simulink model "Proyecto_labII_V1"  (R2025b)
settings: Solver=VariableStepAuto  StartTime=0.0  StopTime=1  RelTol=1e-3
undefined symbols (not defined in the file): gray
libraries: commsequence2 x2, commcrc2 x2, commchan3 x1, commsink2 x1, commcnvcod2 x1
settings Model: Creator=juand  LastModifiedBy=juand

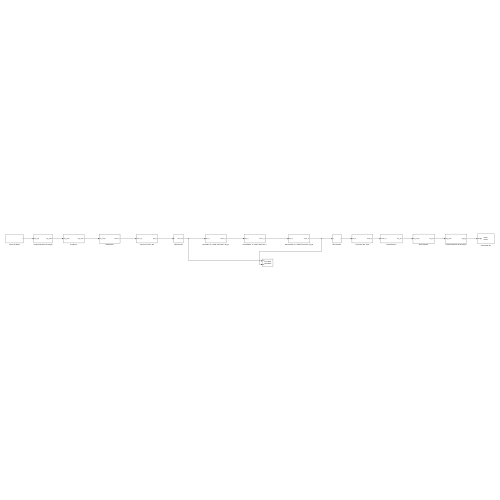
[thumbnail: Simulink's stored preview of the top-level diagram]
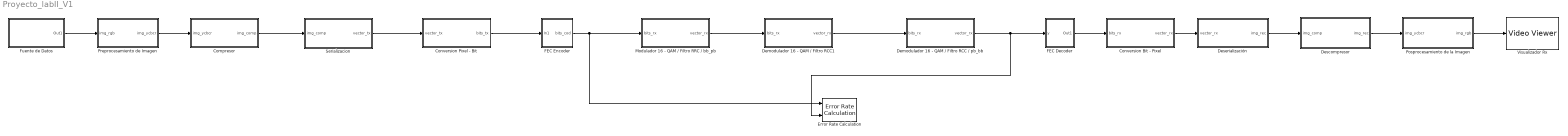
== system Proyecto_labII_V1 ==
  Compresor : Subsystem
  Conversion Bit - Pixel : Subsystem
  Conversion Pixel - Bit : Subsystem
  Demodulador 16 - QAM / Filtro RCC / pb_bb : Subsystem
  Demodulador 16 - QAM / Filtro RCC1 : Subsystem
  Descompresor : Subsystem
  Deserialización : Subsystem
  Error Rate Calculation : commsink2/Error Rate Calculation  N=0  st_delay=0  cp_mode=Entire frame  subframe=[]  PMode=Workspace  WsName=ber_out  RsMode2=off  stop=off  numErr=100  maxBits=1e6
  "FEC Decoder " : Subsystem
  FEC Encoder : Subsystem
  Fuente de Datos : Subsystem
  Modulador 16 - QAM / Filtro RRC / bb_pb : Subsystem
  Posprocesamiento de la Imagen : Subsystem
  Preprocesamiento de Imagen : Subsystem
  Serializacion : Subsystem
  Visualizador Rx : VideoViewer  colormapValue=gray(256)  FigPos=[21 783 890 663]  OpenAtMdlStart=off
  wires:
  Fuente de Datos/1(Out1) -> Preprocesamiento de Imagen/1(img_rgb)
  Preprocesamiento de Imagen/1(img_ycbcr) -> Compresor/1(img_ycbcr)
  Compresor/1(img_comp) -> Serializacion/1(img_comp)
  Deserialización/1(img_rec) -> Descompresor/1(img_comp)
  Descompresor/1(img_rec) -> Posprocesamiento de la Imagen/1(img_ycbcr)
  Serializacion/1(vector_tx) -> Conversion Pixel - Bit/1(vector_tx)
  Conversion Bit - Pixel/1(vector_rx) -> Deserialización/1(vector_rx)
  Posprocesamiento de la Imagen/1(img_rgb) -> Visualizador Rx/1
  Conversion Pixel - Bit/1(bits_tx) -> FEC Encoder/1(In1)
  "FEC Decoder "/1(Out1) -> Conversion Bit - Pixel/1(bits_rx)
  Demodulador 16 - QAM / Filtro RCC / pb_bb/1(vector_rx) -> Error Rate Calculation/2, "FEC Decoder "/1(y)
  FEC Encoder/1(bits_cod) -> Error Rate Calculation/1, Modulador 16 - QAM / Filtro RRC / bb_pb/1(bits_rx)
  Modulador 16 - QAM / Filtro RRC / bb_pb/1(vector_rx) -> Demodulador 16 - QAM / Filtro RCC1/1(bits_rx)
  Demodulador 16 - QAM / Filtro RCC1/1(vector_rx) -> Demodulador 16 - QAM / Filtro RCC / pb_bb/1(bits_rx)

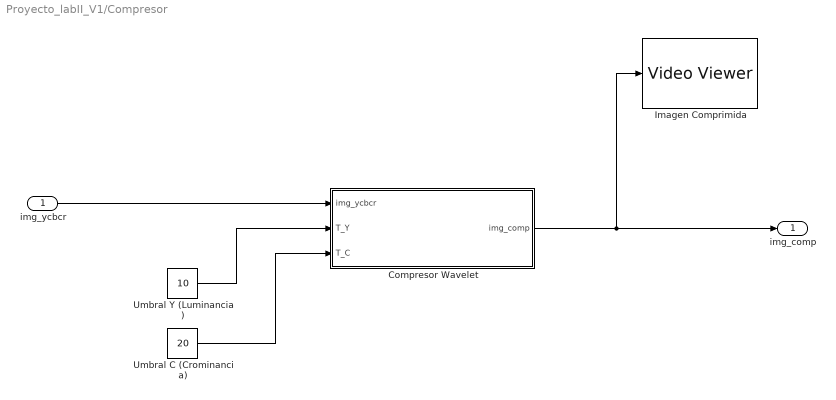
== system Proyecto_labII_V1/Compresor ==
  img_ycbcr : Inport
  Compresor Wavelet : MATLAB Function  TreatAsAtomicUnit=on
  Imagen Comprimida : VideoViewer  colormapValue=gray(256)  FigPos=[1 910 1536 813]  OpenAtMdlStart=off
  Umbral C (Crominancia) : Constant  Value=20
  Umbral Y (Luminancia) : Constant  Value=10
  img_comp : Outport
  wires:
  Compresor Wavelet/1(img_comp) -> Imagen Comprimida/1, img_comp/1
  Umbral C (Crominancia)/1 -> Compresor Wavelet/3(T_C)
  Umbral Y (Luminancia)/1 -> Compresor Wavelet/2(T_Y)
  img_ycbcr/1 -> Compresor Wavelet/1(img_ycbcr)

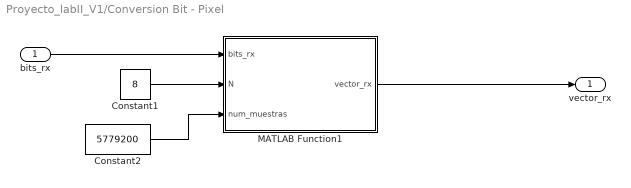
== system Proyecto_labII_V1/Conversion Bit - Pixel ==
  bits_rx : Inport
  Constant1 : Constant  Value=8
  Constant2 : Constant  Value=5779200
  MATLAB Function1 : MATLAB Function  TreatAsAtomicUnit=on
  vector_rx : Outport
  wires:
  Constant1/1 -> MATLAB Function1/2(N)
  bits_rx/1 -> MATLAB Function1/1(bits_rx)
  Constant2/1 -> MATLAB Function1/3(num_muestras)
  MATLAB Function1/1(vector_rx) -> vector_rx/1

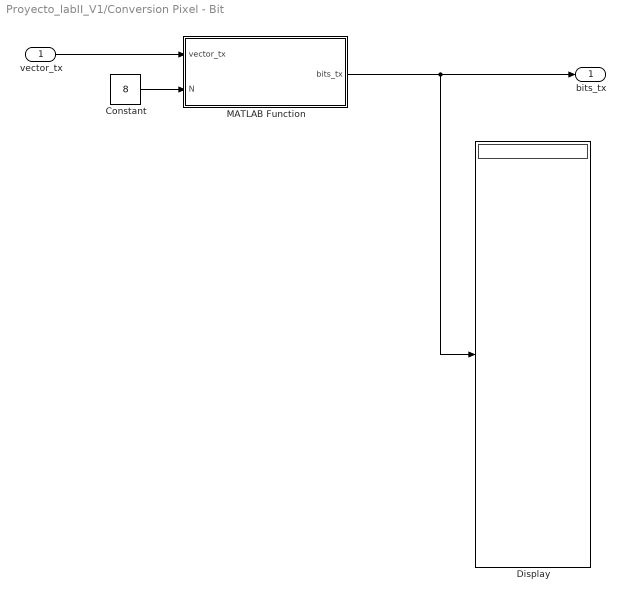
== system Proyecto_labII_V1/Conversion Pixel - Bit ==
  vector_tx : Inport
  Constant : Constant  Value=8
  Display : Display
  MATLAB Function : MATLAB Function  TreatAsAtomicUnit=on
  bits_tx : Outport
  wires:
  Constant/1 -> MATLAB Function/2(N)
  vector_tx/1 -> MATLAB Function/1(vector_tx)
  MATLAB Function/1(bits_tx) -> Display/1, bits_tx/1

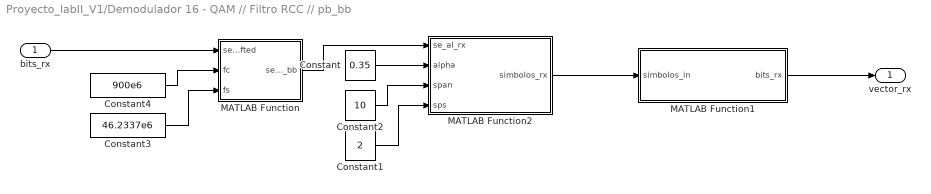
== system Proyecto_labII_V1/Demodulador 16 - QAM // Filtro RCC // pb_bb ==
  bits_rx : Inport
  Constant : Constant  Value=0.35
  Constant1 : Constant  Value=2
  Constant2 : Constant  Value=10
  Constant3 : Constant  Value=46.2337e6
  Constant4 : Constant  Value=900e6
  MATLAB Function : MATLAB Function  TreatAsAtomicUnit=on
  MATLAB Function1 : MATLAB Function  TreatAsAtomicUnit=on
  MATLAB Function2 : MATLAB Function  TreatAsAtomicUnit=on
  vector_rx : Outport
  wires:
  MATLAB Function1/1(bits_rx) -> vector_rx/1
  MATLAB Function2/1(simbolos_rx) -> MATLAB Function1/1(simbolos_in)
  bits_rx/1 -> MATLAB Function/1(senal_shifted)
  Constant1/1 -> MATLAB Function2/4(sps)
  Constant/1 -> MATLAB Function2/2(alpha)
  Constant2/1 -> MATLAB Function2/3(span)
  MATLAB Function/1(senal_bb) -> MATLAB Function2/1(se_al_rx)
  Constant4/1 -> MATLAB Function/2(fc)
  Constant3/1 -> MATLAB Function/3(fs)

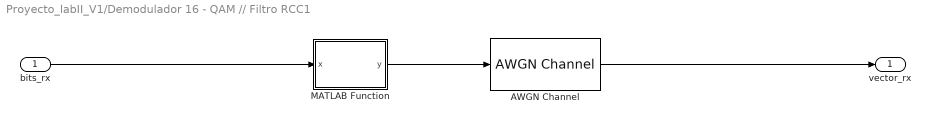
== system Proyecto_labII_V1/Demodulador 16 - QAM // Filtro RCC1 ==
  bits_rx : Inport
  AWGN Channel : commchan3/AWGN Channel  LegacyMode=off  NoiseMethod="Signal to noise ratio  (SNR)"  noiseMode="Signal to noise ratio  (SNR)"  EbNo=EbN0  EsNo=10  SNR=10  BitsPerSymbol=4  SignalPower=1  SpecifySymbolPeriod=off  SamplesPerSymbol=10  SymbolPeriod=1  VarianceSource=Parameter  Variance=1  RandomStream=Global stream  Seed=67  SimulateUsing=Code generation
  MATLAB Function : MATLAB Function  TreatAsAtomicUnit=on
  vector_rx : Outport
  wires:
  AWGN Channel/1 -> vector_rx/1
  MATLAB Function/1(y) -> AWGN Channel/1
  bits_rx/1 -> MATLAB Function/1(x)

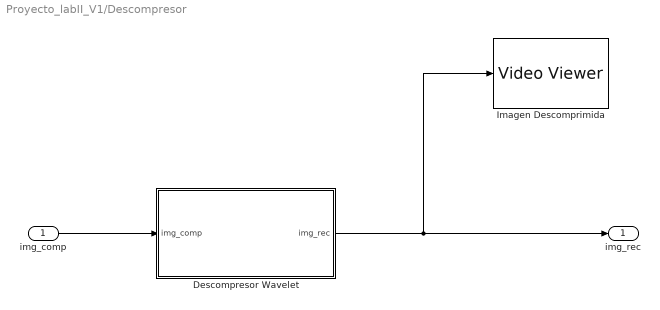
== system Proyecto_labII_V1/Descompresor ==
  img_comp : Inport
  Descompresor Wavelet : MATLAB Function  TreatAsAtomicUnit=on
  Imagen Descomprimida : VideoViewer  colormapValue=gray(256)  FigPos=[1 910 1536 813]  OpenAtMdlStart=off
  img_rec : Outport
  wires:
  Descompresor Wavelet/1(img_rec) -> Imagen Descomprimida/1, img_rec/1
  img_comp/1 -> Descompresor Wavelet/1(img_comp)

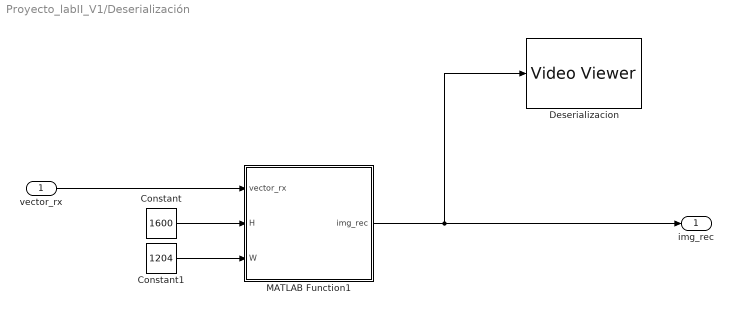
== system Proyecto_labII_V1/Deserialización ==
  vector_rx : Inport
  Constant : Constant  Value=1600
  Constant1 : Constant  Value=1204
  Deserializacion : VideoViewer  FigPos=[559 631 418 304]  OpenAtMdlStart=off
  MATLAB Function1 : MATLAB Function  TreatAsAtomicUnit=on
  img_rec : Outport
  wires:
  Constant1/1 -> MATLAB Function1/3(W)
  Constant/1 -> MATLAB Function1/2(H)
  MATLAB Function1/1(img_rec) -> Deserializacion/1, img_rec/1
  vector_rx/1 -> MATLAB Function1/1(vector_rx)

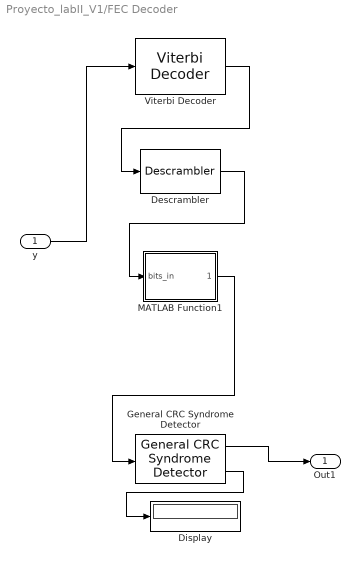
== system Proyecto_labII_V1/FEC Decoder  ==
  y : Inport
  Descrambler : commsequence2/Descrambler  M=2  poly='1 + z^-3 + z^-7'  iniStaSource=Dialog Parameter  ini_sta=[0 0 0 0 0 0 0]  resetViaPort=off
  Display : Display
  General CRC Syndrome Detector : commcrc2/General CRC Syndrome Detector  genPoly='z^16 + z^12 + z^5 + 1'  iniStates=0  directMethod=off  reflectInputBytes=off  reflectChecksums=off  finalXOR=0  numChecksums=1
  MATLAB Function1 : MATLAB Function  TreatAsAtomicUnit=on
  Viterbi Decoder : commcnvcod2/Viterbi Decoder  trellis=poly2trellis(7, [171 133])  isPunctured=off  punctureVector=[1; 1; 0; 1; 0; 1]  erasures=off  dectype=Hard decision  nsdecb=4  runSigValErrCheck=off  tbdepth=35  opmode=Truncated  reset=off  delayedResetAction=on  smWordLength=16  outDataType=double
      settings: LibrarySourceBlock=commhdlcnvcod/Viterbi Decoder
  Out1 : Outport
  wires:
  MATLAB Function1/1(bits_out) -> General CRC Syndrome Detector/1
  Descrambler/1 -> MATLAB Function1/1(bits_in)
  General CRC Syndrome Detector/2 -> Display/1
  Viterbi Decoder/1 -> Descrambler/1
  y/1 -> Viterbi Decoder/1
  General CRC Syndrome Detector/1 -> Out1/1

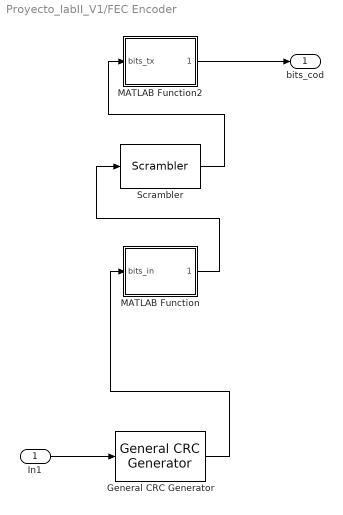
== system Proyecto_labII_V1/FEC Encoder ==
  In1 : Inport
  General CRC Generator : commcrc2/General CRC Generator  genPoly='z^16 + z^12 + z^5 + 1'  iniStates=0  directMethod=off  reflectInputBytes=off  reflectChecksums=off  finalXOR=0  numChecksums=1
  MATLAB Function : MATLAB Function  TreatAsAtomicUnit=on
  MATLAB Function2 : MATLAB Function  TreatAsAtomicUnit=on
  Scrambler : commsequence2/Scrambler  M=2  poly='1 + z^-3 + z^-7'  iniStaSource=Dialog Parameter  ini_sta=[0 0 0 0 0 0 0]  resetViaPort=off
  bits_cod : Outport
  wires:
  General CRC Generator/1 -> MATLAB Function/1(bits_in)
  MATLAB Function2/1(bits_cod) -> bits_cod/1
  MATLAB Function/1(bits_int) -> Scrambler/1
  Scrambler/1 -> MATLAB Function2/1(bits_tx)
  In1/1 -> General CRC Generator/1

== system Proyecto_labII_V1/Fuente de Datos ==
  Fuente de Imagen : FromWorkspace  VariableName=img_ts  SampleTime=1  Interpolate=off  ZeroCross=off  OutputAfterFinalValue=Holding final value
  Visualizador de Imagen en Tx : VideoViewer  FigPos=[559 631 418 304]  OpenAtMdlStart=off
  Out1 : Outport
  wires:
  Fuente de Imagen/1 -> Out1/1, Visualizador de Imagen en Tx/1

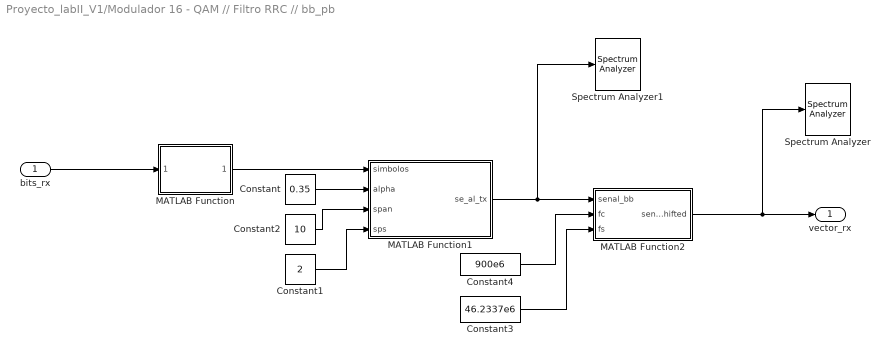
== system Proyecto_labII_V1/Modulador 16 - QAM // Filtro RRC // bb_pb ==
  bits_rx : Inport
  Constant : Constant  Value=0.35
  Constant1 : Constant  Value=2
  Constant2 : Constant  Value=10
  Constant3 : Constant  Value=46.2337e6
  Constant4 : Constant  Value=900e6
  MATLAB Function : MATLAB Function  TreatAsAtomicUnit=on
  MATLAB Function1 : MATLAB Function  TreatAsAtomicUnit=on
  MATLAB Function2 : MATLAB Function  TreatAsAtomicUnit=on
  Spectrum Analyzer : SpectrumAnalyzer  WindowPosition=[482.000000,195.000000,1008.000000,500.000000,]  ScopeFrameLocation=window  WindowInvariantSamplesPerUpdate=on  Span=46233656  StartFrequency=-23116828  StopFrequency=23116828  YLimits=[-85.7412 17.7593]  SelectedToolstripTab=spectrumAnalyzerToolstrip.channelMeasurementsTab
  Spectrum Analyzer1 : SpectrumAnalyzer  ScopeFrameLocation=window  WindowInvariantSamplesPerUpdate=on  Span=46233656  StartFrequency=-23116828  StopFrequency=23116828  YLimits=[-85.7412 17.7593]  SelectedToolstripTab=spectrumAnalyzerToolstrip.channelMeasurementsTab
  vector_rx : Outport
  wires:
  bits_rx/1 -> MATLAB Function/1(bits_cod)
  MATLAB Function/1(simbolos) -> MATLAB Function1/1(simbolos)
  Constant/1 -> MATLAB Function1/2(alpha)
  Constant1/1 -> MATLAB Function1/4(sps)
  Constant2/1 -> MATLAB Function1/3(span)
  MATLAB Function1/1(se_al_tx) -> Spectrum Analyzer1/1, MATLAB Function2/1(senal_bb)
  MATLAB Function2/1(senal_shifted) -> Spectrum Analyzer/1, vector_rx/1
  Constant4/1 -> MATLAB Function2/2(fc)
  Constant3/1 -> MATLAB Function2/3(fs)

== system Proyecto_labII_V1/Posprocesamiento de la Imagen ==
  img_ycbcr : Inport
  Conversión YCbCr→RGB : MATLAB Function  TreatAsAtomicUnit=on
  Posprocesamiento de la Imagen : VideoViewer  colormapValue=gray(256)  FigPos=[1 910 1536 813]  OpenAtMdlStart=off
  img_rgb : Outport
  wires:
  Conversión YCbCr→RGB/1(img_rgb) -> Posprocesamiento de la Imagen/1, img_rgb/1
  img_ycbcr/1 -> Conversión YCbCr→RGB/1(img_ycbcr)

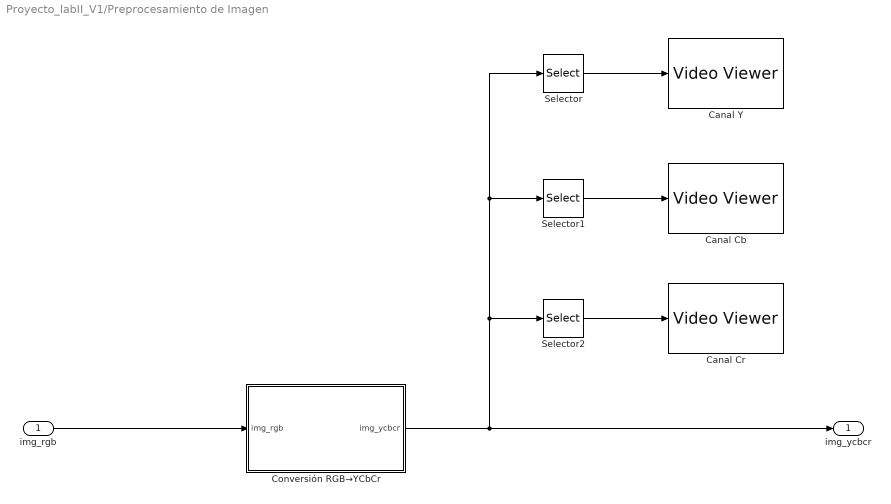
== system Proyecto_labII_V1/Preprocesamiento de Imagen ==
  img_rgb : Inport
  Canal Cb : VideoViewer  colormapValue=gray(256)  FigPos=[559 631 418 304]  OpenAtMdlStart=off
  Canal Cr : VideoViewer  colormapValue=gray(256)  FigPos=[559 631 418 304]  OpenAtMdlStart=off
  Canal Y : VideoViewer  colormapValue=gray(256)  FigPos=[1 910 1536 813]  OpenAtMdlStart=off
  Conversión RGB→YCbCr : MATLAB Function  TreatAsAtomicUnit=on
  Selector : Selector  NumberOfDimensions=3  InputPortWidth=3  IndexOptions=Select all,Select all,Index vector (dialog)  Indices=[1 3],1,1  OutputSizes=1,1,1
  Selector1 : Selector  NumberOfDimensions=3  InputPortWidth=3  IndexOptions=Select all,Select all,Index vector (dialog)  Indices=[1 3],1,2  OutputSizes=1,1,1
  Selector2 : Selector  NumberOfDimensions=3  InputPortWidth=3  IndexOptions=Select all,Select all,Index vector (dialog)  Indices=[1 3],1,3  OutputSizes=1,1,1
  img_ycbcr : Outport
  wires:
  Conversión RGB→YCbCr/1(img_ycbcr) -> img_ycbcr/1, Selector2/1, Selector/1, Selector1/1
  Selector2/1 -> Canal Cr/1
  Selector/1 -> Canal Y/1
  Selector1/1 -> Canal Cb/1
  img_rgb/1 -> Conversión RGB→YCbCr/1(img_rgb)

== system Proyecto_labII_V1/Serializacion ==
  img_comp : Inport
  Display : Display
  MATLAB Function : MATLAB Function  TreatAsAtomicUnit=on
  vector_tx : Outport
  wires:
  img_comp/1 -> MATLAB Function/1(img_comp)
  MATLAB Function/1(vector_tx) -> Display/1, vector_tx/1

== matlab function Proyecto_labII_V1/Posprocesamiento de la Imagen/Conversión YCbCr→RGB ==
  data: img_ycbcr input size=[1600 1204 3]; img_rgb output size=[1600 1204 3]
function img_rgb = bloque3_ycbcr_a_rgb(img_ycbcr)
%#codegen
% BLOQUE 3 - POSTPROCESAMIENTO (Rx): YCbCr → RGB
% Va dentro del MATLAB Function block en Simulink.
%
% ENTRADA:
%   img_ycbcr : imagen YCbCr, uint8, H x W x 3
%               (:,:,1) = Y   luminancia
%               (:,:,2) = Cb  diferencia azul  (centro=128)
%               (:,:,3) = Cr  diferencia rojo  (centro=128)
%
% SALIDA:
%   img_rgb   : imagen RGB reconstruida, uint8, H x W x 3

    % --- Extraer canales y convertir a double ---
    Y_d  = double(img_ycbcr(:,:,1));
    Cb_d = double(img_ycbcr(:,:,2)) - 128.0;
    Cr_d = double(img_ycbcr(:,:,3)) - 128.0;

    % --- Transformación inversa YCbCr → RGB (ITU-R BT.601, full range) ---
    %
    % [ R ]   [ 1.0000   0.0000   1.4020 ] [ Y        ]
    % [ G ] = [ 1.0000  -0.3441  -0.7141 ] [ Cb - 128 ]
    % [ B ]   [ 1.0000   1.7720   0.0000 ] [ Cr - 128 ]
    %
    R_d = Y_d                  + 1.4020 * Cr_d;
    G_d = Y_d - 0.3441 * Cb_d - 0.7141 * Cr_d;
    B_d = Y_d + 1.7720 * Cb_d;

    % --- Clip + conversión a uint8 ---
    R = uint8(max(0, min(255, R_d)));
    G = uint8(max(0, min(255, G_d)));
    B = uint8(max(0, min(255, B_d)));

    % --- Reconstruir imagen RGB ---
    img_rgb = cat(3, R, G, B);
end

== matlab function Proyecto_labII_V1/Modulador 16 - QAM // Filtro RRC // bb_pb/MATLAB Function ==
  data: bits_cod input; simbolos output
function simbolos = bloque_modulador_16qam(bits_cod)
%#codegen
    span = int32(20);  % ← era 10, ahora 20 (span*sps)

    N_bits = length(bits_cod);
    resto  = mod(N_bits, 4);
    if resto ~= 0
        bits_cod = [bits_cod; zeros(4-resto, 1)];
        N_bits   = length(bits_cod);
    end

    N_simbolos = N_bits / 4;
    tabla_I  = [-3 -3 -3 -3 -1 -1 -1 -1  1  1  1  1  3  3  3  3];
    tabla_Q  = [ 3  1 -1 -3  3  1 -1 -3  3  1 -1 -3  3  1 -1 -3];
    gray_map = [ 0  1  3  2  4  5  7  6 12 13 15 14  8  9 11 10];

    simbolos_data = complex(zeros(N_simbolos, 1));
    for k = 1:N_simbolos
        idx     = (k-1)*4 + 1;
        b       = bits_cod(idx:idx+3)';
        decimal = b(1)*8 + b(2)*4 + b(3)*2 + b(4);
        sym_idx = gray_map(decimal+1) + 1;
        simbolos_data(k) = (tabla_I(sym_idx) + 1j*tabla_Q(sym_idx)) / sqrt(10);
    end

    padding  = complex(zeros(span, 1));
    simbolos = [simbolos_data; padding];  % 23,116,828 símbolos
end

== matlab function Proyecto_labII_V1/Demodulador 16 - QAM // Filtro RCC // pb_bb/MATLAB Function2 ==
  data: se_al_rx input; simbolos_rx output; alpha input; span input; sps input
function simbolos_rx = rrc_rx_filter(se_al_rx, alpha, span, sps)
%#codegen
    persistent h zi;

    % Entrada: 46233636 muestras
    % Salida:  23116818 símbolos (46233636 / sps)
    N_out = int32(23116818);  % ← corregido: tamaño POST-downsample
    simbolos_rx = complex(zeros(N_out, 1));

    if isempty(h)
        N = span * sps;
        t = (-N/2 : N/2) / sps;
        h = zeros(1, length(t));
        for i = 1:length(t)
            n = t(i);
            if n == 0
                h(i) = (1/sqrt(sps))*(1 - alpha + 4*alpha/pi);
            elseif abs(abs(n) - 1/(4*alpha)) < 1e-10
                h(i) = (alpha/sqrt(2*sps)) * ...
                       ((1+2/pi)*sin(pi/(4*alpha)) + ...
                        (1-2/pi)*cos(pi/(4*alpha)));
            else
                num = sin(pi*n*(1-alpha)) + 4*alpha*n*cos(pi*n*(1+alpha));
                den = pi*n*(1-(4*alpha*n)^2)*sqrt(sps);
                h(i) = num/den;
            end
        end
        h  = h / sqrt(sum(h.^2));
        zi = complex(zeros(length(h)-1, 1));
    end

    % Filtrar con estado
    [y, zi] = filter(h, 1, double(se_al_rx), zi);

    % Downsample: tomar 1 de cada sps muestras → 46233636/2 = 23116818
    for k = int32(1):N_out
        simbolos_rx(k) = y(int32(1) + (k - int32(1)) * int32(sps));
    end
end

== matlab function Proyecto_labII_V1/Demodulador 16 - QAM // Filtro RCC // pb_bb/MATLAB Function1 ==
  data: simbolos_in input; bits_rx output
function bits_rx = bloque_demodulador_16qam(simbolos_in)
%#codegen
    span       = int32(10);
    N_simbolos = int32(23116808);
    N_bits     = N_simbolos * int32(4);
    bits_rx    = zeros(N_bits, 1);

    % Saltar los primeros span símbolos (transitorio del filtro)
    % y tomar exactamente N_simbolos desde ahí ← corrección clave
    simbolos = simbolos_in(span+int32(1) : span+N_simbolos);

    tabla_I      = [-3 -3 -3 -3 -1 -1 -1 -1  1  1  1  1  3  3  3  3];
    tabla_Q      = [ 3  1 -1 -3  3  1 -1 -3  3  1 -1 -3  3  1 -1 -3];
    gray_map     = [ 0  1  3  2  4  5  7  6 12 13 15 14  8  9 11 10];
    gray_map_inv = zeros(1,16);
    for i = 1:16
        gray_map_inv(gray_map(i)+1) = i-1;
    end

    simbolos_rx = simbolos * sqrt(10);

    for k = 1:N_simbolos
        I_rx     = real(simbolos_rx(k));
        Q_rx     = imag(simbolos_rx(k));
        dist_min = inf;
        idx_min  = 1;
        for m = 1:16
            dist = (I_rx-tabla_I(m))^2 + (Q_rx-tabla_Q(m))^2;
            if dist < dist_min
                dist_min = dist;
                idx_min  = m;
            end
        end
        decimal          = gray_map_inv(idx_min);
        idx_out          = (k-1)*4 + 1;
        bits_rx(idx_out)   = bitget(uint8(decimal),4);
        bits_rx(idx_out+1) = bitget(uint8(decimal),3);
        bits_rx(idx_out+2) = bitget(uint8(decimal),2);
        bits_rx(idx_out+3) = bitget(uint8(decimal),1);
    end
end

== matlab function Proyecto_labII_V1/Modulador 16 - QAM // Filtro RRC // bb_pb/MATLAB Function2 ==
  data: senal_bb input; senal_shifted output; fc input; fs input
function senal_shifted = upconvert(senal_bb, fc, fs)
%#codegen
% Desplazamiento en frecuencia: traslada el espectro de f=0 a f=fc
% Equivalente digital de lo que hace el mezclador RF de la USRP
    N = int32(46233656);
    n = (0:double(N)-1)';
    senal_shifted = senal_bb .* exp(1j*2*pi*(fc/fs)*n);
end

== matlab function Proyecto_labII_V1/Demodulador 16 - QAM // Filtro RCC // pb_bb/MATLAB Function ==
  data: senal_shifted input; senal_bb output; fc input; fs input
function senal_bb = downconvert(senal_shifted, fc, fs)
%#codegen
% Desplazamiento inverso: traslada el espectro de f=fc a f=0
    N = int32(46233656);
    n = (0:double(N)-1)';
    senal_bb = senal_shifted .* exp(-1j*2*pi*(fc/fs)*n);
end

== matlab function Proyecto_labII_V1/Demodulador 16 - QAM // Filtro RCC1/MATLAB Function ==
  data: x input; y output
function y = MATLAB_Function(x)
% Canal multitrayecto suave: rayo directo + eco débil

alpha = 0.1;   % Atenuación del rayo reflejado
D = 2;         % Retardo en muestras

x = x(:);

if length(x) <= D
    y = x;
    return;
end

x_delay = [zeros(D,1); x(1:end-D)];

% Normalización para no aumentar demasiado la potencia
y = (x + alpha*x_delay) / sqrt(1 + alpha^2);
end

== matlab function Proyecto_labII_V1/Preprocesamiento de Imagen/Conversión RGB→YCbCr ==
  data: img_rgb input size=[1600 1204 3]; img_ycbcr output size=[1600 1204 3]
function img_ycbcr = bloque2_rgb_a_ycbcr(img_rgb)
%#codegen
% BLOQUE 2 - PREPROCESAMIENTO (Tx): RGB → YCbCr
% Va dentro del MATLAB Function block en Simulink.
%
% ENTRADA:
%   img_rgb   : imagen RGB,   uint8, H x W x 3
%
% SALIDA:
%   img_ycbcr : imagen YCbCr, uint8, H x W x 3
%               (:,:,1) = Y   luminancia
%               (:,:,2) = Cb  diferencia azul  (centro=128)
%               (:,:,3) = Cr  diferencia rojo  (centro=128)

    % --- Extraer canales R, G, B como double ---
    R = double(img_rgb(:,:,1));
    G = double(img_rgb(:,:,2));
    B = double(img_rgb(:,:,3));

    % --- Transformación RGB → YCbCr (ITU-R BT.601, full range) ---
    %
    % [ Y  ]   [ 0.2989   0.5870   0.1140 ] [ R ]   [   0 ]
    % [ Cb ] = [-0.1687  -0.3313   0.5000 ] [ G ] + [ 128 ]
    % [ Cr ]   [ 0.5000  -0.4187  -0.0813 ] [ B ]   [ 128 ]
    %
    Y_d  =  0.2989 * R + 0.5870 * G + 0.1140 * B;
    Cb_d = -0.1687 * R - 0.3313 * G + 0.5000 * B + 128.0;
    Cr_d =  0.5000 * R - 0.4187 * G - 0.0813 * B + 128.0;

    % --- Clip + conversión a uint8 ---
    Y  = uint8(max(0, min(255, Y_d)));
    Cb = uint8(max(0, min(255, Cb_d)));
    Cr = uint8(max(0, min(255, Cr_d)));

    % --- Apilar en un solo stack H x W x 3 ---
    img_ycbcr = cat(3, Y, Cb, Cr);
end

== matlab function Proyecto_labII_V1/Compresor/Compresor Wavelet ==
  data: img_ycbcr input uint8 size=[1600 1204 3]; img_comp output double size=[1600 1204 3]; T_Y input double size=1; T_C input double size=1
function img_comp = bloque_wavelet_tx(img_ycbcr, T_Y, T_C)
%#codegen
% BLOQUE WAVELET Tx - Transformada Haar + Umbralización (3 canales)
%
% ENTRADAS:
%   img_ycbcr : imagen YCbCr, uint8, H x W x 3
%   T_Y       : umbral canal Y  (recomendado: 10)
%   T_C       : umbral Cb y Cr  (recomendado: 20)
%
% SALIDA:
%   img_comp  : imagen comprimida, double, H x W x 3

    [m, n, ~] = size(img_ycbcr);
    m2 = floor(m/2)*2;
    n2 = floor(n/2)*2;

    img_comp = zeros(m2, n2, 3);
    T = [T_Y, T_C, T_C];

    for c = 1:3
        I = double(img_ycbcr(1:m2, 1:n2, c));

        % Haar horizontal
        L = (I(:, 1:2:n2) + I(:, 2:2:n2)) / 2;
        H = (I(:, 1:2:n2) - I(:, 2:2:n2)) / 2;

        % Haar vertical
        LL = (L(1:2:m2,:) + L(2:2:m2,:)) / 2;
        LH = (L(1:2:m2,:) - L(2:2:m2,:)) / 2;
        HL = (H(1:2:m2,:) + H(2:2:m2,:)) / 2;
        HH = (H(1:2:m2,:) - H(2:2:m2,:)) / 2;

        % Umbralización
        LH(abs(LH) < T(c)) = 0;
        HL(abs(HL) < T(c)) = 0;
        HH(abs(HH) < T(c)) = 0;

        img_comp(:,:,c) = [LL, HL; LH, HH];
    end
end

== matlab function Proyecto_labII_V1/Descompresor/Descompresor Wavelet ==
  data: img_comp input double size=[1600 1204 3]; img_rec output uint8 size=[1600 1204 3]
function img_rec = bloque_wavelet_rx(img_comp)
%#codegen
% BLOQUE WAVELET Rx - Transformada Haar Inversa (3 canales)
%
% ENTRADA:
%   img_comp : imagen comprimida, double, H x W x 3
%
% SALIDA:
%   img_rec  : imagen YCbCr reconstruida, uint8, H x W x 3

    [m, n, ~] = size(img_comp);
    m2 = m/2;
    n2 = n/2;

    img_rec = zeros(m, n, 3, 'uint8');

    for c = 1:3

        % Extraer subbandas
        LL = img_comp(1:m2,   1:n2,   c);
        HL = img_comp(1:m2,   n2+1:n, c);
        LH = img_comp(m2+1:m, 1:n2,   c);
        HH = img_comp(m2+1:m, n2+1:n, c);

        % Haar inversa vertical
        L = zeros(m, n2);
        H = zeros(m, n2);

        L(1:2:m,:) = LL + LH;
        L(2:2:m,:) = LL - LH;
        H(1:2:m,:) = HL + HH;
        H(2:2:m,:) = HL - HH;

        % Haar inversa horizontal
        I_rec = zeros(m, n);
        I_rec(:, 1:2:n) = L + H;
        I_rec(:, 2:2:n) = L - H;

        img_rec(:,:,c) = uint8(max(0, min(255, I_rec)));
    end
end

== matlab function Proyecto_labII_V1/Serializacion/MATLAB Function ==
  data: img_comp input double size=[1600 1204 3]; vector_tx output double size=[5779200 1]
function vector_tx = bloque_serializacion(img_comp)
%#codegen
% BLOQUE SERIALIZACIÓN - Imagen 3D → Vector 1D
% Va dentro del MATLAB Function block en Simulink.
%
% ENTRADA:
%   img_comp  : imagen comprimida, double, H x W x 3
%
% SALIDA:
%   vector_tx : vector serializado, double, (H*W*3) x 1

    vector_tx = img_comp(:);
end

== matlab function Proyecto_labII_V1/Deserialización/MATLAB Function1 ==
  data: vector_rx input double size=[5779200 1]; img_rec output double size=[1600 1204 3]; H input double size=1; W input double size=1
function img_rec = bloque_deserializacion(vector_rx, H, W)
%#codegen
% BLOQUE DESERIALIZACIÓN - Vector 1D → Imagen 3D
% Va dentro del MATLAB Function block en Simulink.
%
% ENTRADAS:
%   vector_rx : vector recibido, double, (H*W*3) x 1
%   H         : alto de la imagen  (ej: 1600)
%   W         : ancho de la imagen (ej: 1204)
%
% SALIDA:
%   img_rec   : imagen reconstruida, double, H x W x 3

    img_rec = reshape(vector_rx, H, W, 3);
end

== matlab function Proyecto_labII_V1/Conversion Pixel - Bit/MATLAB Function ==
  data: vector_tx input double size=[5779200 1]; bits_tx output double size=[46233600 1]; N input double size=1
function bits_tx = bloque_pixeles_a_bits(vector_tx, N)

%#codegen
% BLOQUE PÍXELES → BITS (Cuantización uniforme de N bits)
% Va dentro del MATLAB Function block en Simulink.
%
% ENTRADAS:
%   vector_tx : vector serializado, double, (H*W*3) x 1
%   N         : número de bits por muestra (recomendado: 8)
%
% SALIDA:
%   bits_tx   : vector de bits, double, (H*W*3*N) x 1
%               cada muestra se representa con N bits (MSB primero)

    num_muestras = numel(vector_tx);
    niveles      = 2^N - 1;

    % --- Cuantización: escalar al rango [0, 2^N - 1] ---
    % Los valores del wavelet pueden salirse del rango [0,255]
    % se hace clip antes de cuantizar
    val_clip = max(0, min(niveles, round(vector_tx)));
    val_int  = uint16(val_clip);

    % --- Conversión a bits (MSB primero) ---
    bits_tx = zeros(num_muestras * N, 1);

    for i = 1:num_muestras
        for b = 1:N
            % Extraer bit b (MSB = bit N, LSB = bit 1)
            bits_tx((i-1)*N + b) = double(bitget(val_int(i), N - b + 1));
        end
    end
end

== matlab function Proyecto_labII_V1/Conversion Bit - Pixel/MATLAB Function1 ==
  data: bits_rx input double size=[46233600 1]; vector_rx output double size=[5779200 1]; N input double size=1; num_muestras input double size=1
function vector_rx = bloque_bits_a_pixeles(bits_rx, N, num_muestras)
%#codegen
% BLOQUE BITS → PÍXELES (Reconstrucción desde cuantización uniforme)
% Va dentro del MATLAB Function block en Simulink.
%
% ENTRADAS:
%   bits_rx      : vector de bits recibidos, double, (H*W*3*N) x 1
%   N            : número de bits por muestra (debe coincidir con Tx)
%   num_muestras : número total de muestras = H*W*3 (ej: 5779200)
%
% SALIDA:
%   vector_rx    : vector reconstruido, double, (H*W*3) x 1

    vector_rx = zeros(num_muestras, 1);

    for i = 1:num_muestras
        valor = 0;
        for b = 1:N
            % Reconstruir valor desde bits (MSB primero)
            bit = bits_rx((i-1)*N + b);
            valor = valor + bit * 2^(N - b);
        end
        vector_rx(i) = valor;
    end
end

== matlab function Proyecto_labII_V1/FEC Encoder/MATLAB Function ==
  data: bits_in input double size=[46233616 1]; bits_int output double size=[46233616 1]
function bits_int = bloque_interleaver(bits_in)
%#codegen
% INTERLEAVER MATRICIAL
%
% ENTRADA:
%   bits_in  : double, 46233616 x 1
%
% SALIDA:
%   bits_int : double, 46233616 x 1

    filas = 6292;
    cols  = 7348;

    % Escribir por filas (6292x7348), leer por columnas
    matriz   = reshape(bits_in, filas, cols);
    bits_int = reshape(matriz', filas * cols, 1);
end

== matlab function Proyecto_labII_V1/FEC Decoder /MATLAB Function1 ==
  data: bits_in input double size=[46233616 1]; bits_out output double size=[46233616 1]
function bits_out = bloque_deinterleaver(bits_in)
%#codegen
% DEINTERLEAVER MATRICIAL (inverso exacto del Interleaver)
%
% ENTRADA:
%   bits_in  : double, 46233616 x 1
%
% SALIDA:
%   bits_out : double, 46233616 x 1

    filas = 6292;
    cols  = 7348;

    % Escribir por filas (7348x6292), leer por columnas
    % Operación inversa exacta del interleaver
    matriz   = reshape(bits_in, cols, filas);
    bits_out = reshape(matriz', filas * cols, 1);
end

== matlab function Proyecto_labII_V1/FEC Encoder/MATLAB Function2 ==
  data: bits_tx input size=[46233616 1]; bits_cod output size=[92467232 1]
function bits_cod = bloque_codificador_conv(bits_tx)
%#codegen
% CODIFICADOR CONVOLUCIONAL PROPIO
% Tasa 1/2, Constraint Length 7
% Polinomios generadores: [171 133] en octal (estándar NASA)
%
% ENTRADA:
%   bits_tx  : vector de bits, double, (46233616) x 1
%
% SALIDA:
%   bits_cod : bits codificados, double, (92467232) x 1

    % --- Polinomios generadores en binario ---
    g1 = [1 1 1 1 0 0 1];  % 171 octal
    g2 = [1 0 1 1 0 1 1];  % 133 octal

    M = 6;  % Longitud registro = constraint length - 1

    % --- Preasignar salida con tamaño FIJO explícito ---
    bits_cod = zeros(92467232, 1);

    % --- Registro de desplazamiento ---
    registro = zeros(1, M);

    % --- Procesar bit a bit ---
    for i = 1:46233616

        bit_in = bits_tx(i);
        estado = [bit_in, registro];

        % XOR con polinomios
        out1 = mod(sum(estado .* g1), 2);
        out2 = mod(sum(estado .* g2), 2);

        % Guardar salida
        bits_cod(2*i - 1) = out1;
        bits_cod(2*i)     = out2;

        % Desplazar registro
        registro = [bit_in, registro(1:M-1)];
    end
end

== matlab function Proyecto_labII_V1/Modulador 16 - QAM // Filtro RRC // bb_pb/MATLAB Function1 ==
  data: simbolos input; se_al_tx output; alpha input; span input; sps input
function se_al_tx = rrc_tx_filter(simbolos, alpha, span, sps)
%#codegen
    persistent h zi;

    % N_out = N_simbolos * sps = 23116818 * 2
    N_out = int32(46233656);
    se_al_tx = complex(zeros(N_out, 1));

    if isempty(h)
        N = span * sps;
        t = (-N/2 : N/2) / sps;
        h = zeros(1, length(t));
        for i = 1:length(t)
            n = t(i);
            if n == 0
                h(i) = (1/sqrt(sps))*(1 - alpha + 4*alpha/pi);
            elseif abs(abs(n) - 1/(4*alpha)) < 1e-10
                h(i) = (alpha/sqrt(2*sps)) * ...
                       ((1+2/pi)*sin(pi/(4*alpha)) + ...
                        (1-2/pi)*cos(pi/(4*alpha)));
            else
                num = sin(pi*n*(1-alpha)) + 4*alpha*n*cos(pi*n*(1+alpha));
                den = pi*n*(1-(4*alpha*n)^2)*sqrt(sps);
                h(i) = num/den;
            end
        end
        h  = h / sqrt(sum(h.^2));
        zi = complex(zeros(length(h)-1, 1));
    end

    % Upsample: sim_up tiene 46233636, simbolos tiene 23116818
    sim_up = complex(zeros(N_out, 1));
    sim_up(1:sps:end) = double(simbolos); 

    % Filtrar con estado persistente
    [se_al_tx, zi] = filter(h, 1, sim_up, zi);
end
